simulink model "InverseKinematicsIndexFinger"  (Simulink 6.6)
settings: Solver=ode45  StartTime=0.0  StopTime=10.0  RelTol=1e-3
libraries: dspinverses x1
settings Model: Creator=Jadav Das  LastModifiedBy=Jadav Das

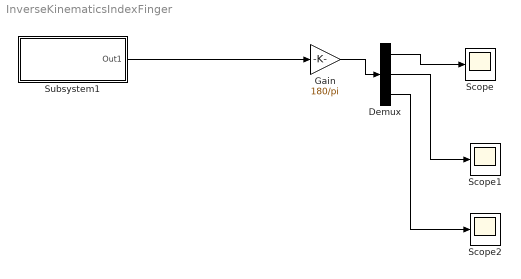
== system InverseKinematicsIndexFinger ==
  Demux : Demux  Outputs=3
  Gain : Gain  Gain=180/pi
  Scope : Scope
      settings: YMin=-0.013  YMax=0.01
  Scope1 : Scope
      settings: YMin=-0.00025  YMax=0.00025
  Scope2 : Scope
      settings: YMin=-0.00025  YMax=0.00025  SaveName=ScopeData2
  Subsystem1 : Subsystem
  wires:
  Gain/1 -> Demux/1
  Demux/1 -> Scope/1
  Demux/2 -> Scope1/1
  Demux/3 -> Scope2/1
  Subsystem1/1(Out1) -> Gain/1

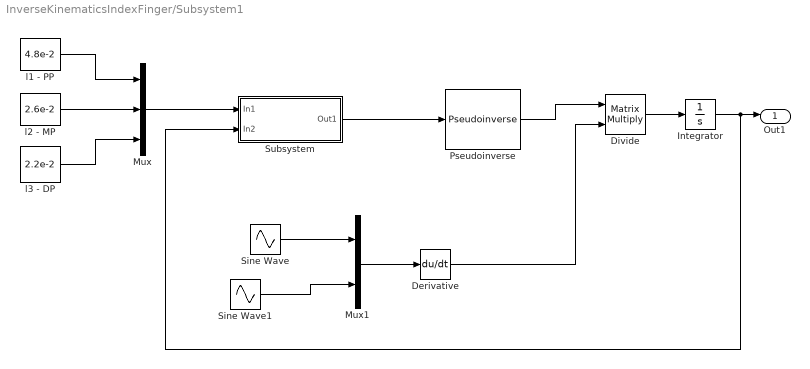
== system InverseKinematicsIndexFinger/Subsystem1 ==
  Derivative : Derivative
  Divide : Product  Inputs=**  Multiplication=Matrix(*)  OutScaling=2^-10
  Integrator : Integrator
  Mux : Mux  Inputs=3
  Mux1 : Mux  Inputs=2
  Pseudoinverse : dspinverses/Pseudoinverse  wanterr=off
  Sine Wave : Sin  Amplitude=4  SampleTime=0
  Sine Wave1 : Sin  Amplitude=3  SampleTime=0
  Subsystem : Subsystem
  l1 - PP : Constant  Value=4.8e-2
  l2 - MP : Constant  Value=2.6e-2
  l3 - DP : Constant  Value=2.2e-2
  Out1 : Outport
  wires:
  l1 - PP/1 -> Mux/1
  l2 - MP/1 -> Mux/2
  l3 - DP/1 -> Mux/3
  Mux/1 -> Subsystem/1(In1)
  Subsystem/1(Out1) -> Pseudoinverse/1
  Pseudoinverse/1 -> Divide/1
  Sine Wave/1 -> Mux1/1
  Sine Wave1/1 -> Mux1/2
  Mux1/1 -> Derivative/1
  Divide/1 -> Integrator/1
  Integrator/1 -> Subsystem/2(In2), Out1/1
  Derivative/1 -> Divide/2

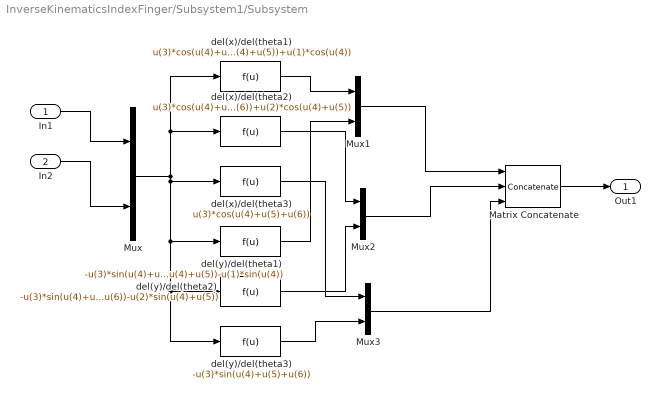
== system InverseKinematicsIndexFinger/Subsystem1/Subsystem ==
  In1 : Inport
  In2 : Inport  Port=2
  Matrix Concatenate : Concatenate  NumInputs=3  Mode=Multidimensional array  ConcatenateDimension=2
  Mux{,1..3} (4 alike) : Mux  Inputs=2
  del(x)/del(theta1) : Fcn  Expr=u(3)*cos(u(4)+u(5)+u(6))+u(2)*cos(u(4)+u(5))+u(1)*cos(u(4))
  del(x)/del(theta2) : Fcn  Expr=u(3)*cos(u(4)+u(5)+u(6))+u(2)*cos(u(4)+u(5))
  del(x)/del(theta3) : Fcn  Expr=u(3)*cos(u(4)+u(5)+u(6))
  del(y)/del(theta1) : Fcn  Expr=-u(3)*sin(u(4)+u(5)+u(6))-u(2)*sin(u(4)+u(5))-u(1)*sin(u(4))
  del(y)/del(theta2) : Fcn  Expr=-u(3)*sin(u(4)+u(5)+u(6))-u(2)*sin(u(4)+u(5))
  del(y)/del(theta3) : Fcn  Expr=-u(3)*sin(u(4)+u(5)+u(6))
  Out1 : Outport
  wires:
  In1/1 -> Mux/1
  In2/1 -> Mux/2
  Mux/1 -> del(x)/del(theta1)/1, del(x)/del(theta2)/1, del(x)/del(theta3)/1, del(y)/del(theta1)/1, del(y)/del(theta2)/1, del(y)/del(theta3)/1
  Matrix Concatenate/1 -> Out1/1
  del(x)/del(theta1)/1 -> Mux1/1
  del(y)/del(theta1)/1 -> Mux1/2
  del(x)/del(theta2)/1 -> Mux2/1
  del(x)/del(theta3)/1 -> Mux3/1
  del(y)/del(theta2)/1 -> Mux2/2
  del(y)/del(theta3)/1 -> Mux3/2
  Mux1/1 -> Matrix Concatenate/1
  Mux2/1 -> Matrix Concatenate/2
  Mux3/1 -> Matrix Concatenate/3
